simulink model "gm_minutiaeextraction_21821"  (R2018b)
settings: Solver=FixedStepDiscrete  StartTime=0.0  StopTime=10  RelTol=1e-3
undefined symbols (not defined in the file or in its folder): gray
libraries: hdlsllib x4, visionsources x1, dspmtrx3 x1
(part 4 of 7)

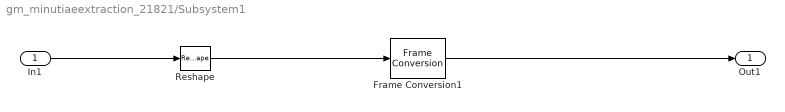
== system gm_minutiaeextraction_21821/Subsystem1 ==
  In1 : Inport
  Frame Conversion1 : FrameConversion  OutFrame=Sample-based
  Reshape : Reshape
  Out1 : Outport
  wires:
  In1/1 -> Reshape/1
  Reshape/1 -> Frame Conversion1/1
  Frame Conversion1/1 -> Out1/1

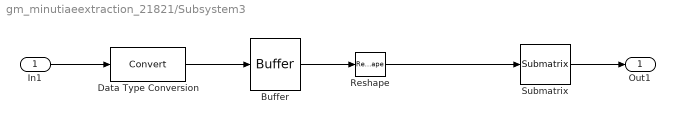
== system gm_minutiaeextraction_21821/Subsystem3 ==
  In1 : Inport
  Buffer : Buffer  N=8192  OutputFrames=off
  Data Type Conversion : DataTypeConversion
  Reshape : Reshape  OutputDimensionality=Customize  OutputDimensions=[128,64]
  Submatrix : dspmtrx3/Submatrix  RowSpan=Range of rows  RowStartMode=First  RowStartIndex=1  RowEndMode=Last  RowEndIndex=1  ColSpan=Range of columns  ColStartMode=First  ColStartIndex=1  ColEndMode=Last  ColEndIndex=1
  Out1 : Outport
  wires:
  In1/1 -> Data Type Conversion/1
  Submatrix/1 -> Out1/1
  Reshape/1 -> Submatrix/1
  Buffer/1 -> Reshape/1
  Data Type Conversion/1 -> Buffer/1

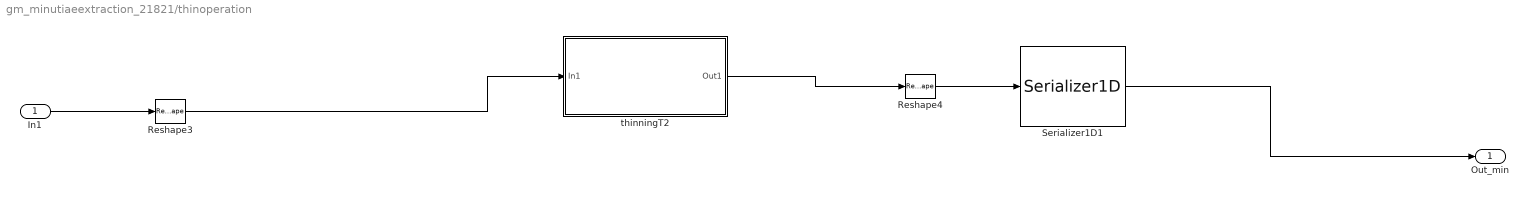
== system gm_minutiaeextraction_21821/thinoperation ==
  In1 : Inport
  Reshape3 : Reshape  OutputDimensionality=Customize  OutputDimensions=[128,64]
  Reshape4 : Reshape  OutputDimensionality=Column vector (2-D)  OutputDimensions=[128,64]
  Serializer1D1 : hdlsllib/HDL Operations/Serializer1D  Ratio=1  IdleCycles=0  validIn=off  startOut=off  validOut=off  inputDataDimensions=-1  inputSampleTime=-1  inputSignalType=auto
      settings: SourceProductName=HDL Coder  SourceProductBaseCode=HD
  thinningT2 : Subsystem  TreatAsAtomicUnit=on
  Out_min : Outport
  wires:
  Reshape4/1 -> Serializer1D1/1
  In1/1 -> Reshape3/1
  Serializer1D1/1 -> Out_min/1
  Reshape3/1 -> thinningT2/1(In1)
  thinningT2/1(Out1) -> Reshape4/1
